simulink model "HVModAL_Fahrzeugmodell"  (R2015b)
settings: Solver=ode1  StartTime=0  StopTime=drp.driving_cycle.tstop  FixedStep=sim_params.Ts  RelTol=1e-5
PreLoadFcn:
  | % Add paths
  | addpath data
  | addpath(genpath('library'))
StartFcn:
  | Simulation.StartTime = tic;
StopFcn:
  | Simulation.DurationTime = toc(Simulation.StartTime);
undefined symbols (not defined in the file or in its folder): Batteries, BMS, BMS_Bat_, C_Nenn_DCDC1, C_Nenn_DCDC2, d2d, DC, DCDC_Converter_efficiency, DcDc_Converters, Dcl, drp, drv, elm, gen, gin, Hdc, hdc, HV, hvb, Hvb, ice, ldc, lib_dcl, lib_hdc, lib_hvb, lib_veh, Link, lossestable, mask_LUT_OCV, mask_LUT_OCV_SOC, mask_LUT_OCV_Temperature, mask_LUT_R, mask_LUT_Rs, mask_LUT_Rs_SOC, mask_LUT_Rs_Temperature, sim_params, speedvec, torquevec, tri, veh, Veh, Vehicle_Chassis
libraries: simulink x29, lib_tri_modules x7, lib_hdc_module x5, lib_gearbox x4, lib_hvb_battery_pack x3, cstblocks x3, PowerLimitBlock x2, MultiCellLibrary x2, lib_aux x1, lib_drv x1, lib_gen x1, lib_elm x1
(part 2 of 7)

== system HVModAL_Fahrzeugmodell/Visualization (Vis) ==
  note: Block Data
  note: Overview
  note: Extended Scopes
  Model Info : simulink/Model-Wide Utilities/Model Info  Frame=on  DisplayStringWithTags=|  HorizontalTextAlignment=Center  LeftAlignmentValue=0.5  SourceBlockDiagram=HVModAL_Fahrzeugmodell  TagMaxNumber=20
      | Last modified
      | %<LastModificationDate>
      | 
      | Model Version
      | %<ModelVersion>
  Show Extended Scope on/off : Constant  Value=sim_params.showextendedscopes
  Speed : Subsystem
  Speed Scope : Scope  NumInputPorts=3
  Subsystem1 : Subsystem
  wires:
  Speed/2(v_actual(km/h)) -> Speed Scope/2  "v_actual(km/h)"
  Speed/1(v_cycle(km/h)) -> Speed Scope/1  "v_cycle(km/h)"
  Speed/3(v_deviation(km/h)) -> Speed Scope/3  "v_deviation(km/h)"
  Show Extended Scope on/off/1 -> ?

== system HVModAL_Fahrzeugmodell/DC-Link (Dcl)/Dcl Voltage Calculation ==
  P : Inport
  Sum of Elements1 : Sum  Inputs=+  SaturateOnIntegerOverflow=on
  Terminator : Terminator
  Dcl_U : Outport
  wires:
  [Dcl_U] -> Sum of Elements1/1
  P/1 -> Terminator/1
  Sum of Elements1/1 -> Dcl_U/1

== system HVModAL_Fahrzeugmodell/Energy Manager (Emg)/Aux Control ==
  Tri_BusPW : Inport
  Hdc_BusPW : Inport  Port=2
  Hvb_BusPW : Inport  Port=3
  Tri_BusSW : Inport  Port=4
  Bus Creator1 : BusCreator  Inputs=3
  Bus Selector : BusSelector  OutputSignals=Tri_P_losses_vec
  Bus Selector1 : BusSelector  OutputSignals=PB_Bat1.Total_Dissipation_Power_W,PB_Bat2.Total_Dissipation_Power_W,PB_Bat3.Total_Dissipation_Power_W,PB_Bat4.Total_Dissipation_Power_W,PB_Bat5.Total_Dissipation_Power_W
  Bus Selector2 : BusSelector  OutputSignals=Hdc_P_losses_vec
  Bus Selector3 : BusSelector  OutputSignals=Elm_P_losses_vec
  Emg_auxControl_hvac : Constant  Value=0
  Emg_auxControl_permanentLoad : Constant
  Sum : Sum  Inputs=++++
  Sum of Elements : Sum  Inputs=+
  Sum of Elements1 : Sum  Inputs=+
  Sum of Elements2 : Sum  Inputs=+
  Sum1 : Sum  Inputs=+++++
  Unit Delay : UnitDelay  SampleTime=sim_params.Ts
  Emg_auxControl_BusSW : Outport
  wires:
  Bus Creator1/1 -> Emg_auxControl_BusSW/1  "Emg_auxControl_BusSW"
  Emg_auxControl_permanentLoad/1 -> Bus Creator1/1  "Emg_auxControl_permanentLoad"
  Emg_auxControl_hvac/1 -> Bus Creator1/2  "Emg_auxControl_hvac"
  Tri_BusPW/1 -> Bus Selector/1
  Hdc_BusPW/1 -> Bus Selector2/1
  Hvb_BusPW/1 -> Bus Selector1/1
  Tri_BusSW/1 -> Bus Selector3/1
  Bus Selector/1 -> Sum of Elements/1  "<Tri_P_losses_vec>"
  Bus Selector2/1 -> Sum of Elements1/1  "<Hdc_P_losses_vec>"
  Bus Selector3/1 -> Sum of Elements2/1  "<Elm_P_losses_vec>"
  Sum/1 -> Unit Delay/1
  Unit Delay/1 -> Bus Creator1/3  "Emg_Cooling_demand"
  Sum of Elements/1 -> Sum/1
  Sum of Elements1/1 -> Sum/3
  Bus Selector1/1 -> Sum1/1  "<Total_Dissipation_Power_W>"
  Bus Selector1/2 -> Sum1/2  "<Total_Dissipation_Power_W>"
  Bus Selector1/3 -> Sum1/3  "<Total_Dissipation_Power_W>"
  Bus Selector1/5 -> Sum1/5  "<Total_Dissipation_Power_W>"
  Bus Selector1/4 -> Sum1/4  "<Total_Dissipation_Power_W>"
  Sum1/1 -> Sum/2
  Sum of Elements2/1 -> Sum/4

== system HVModAL_Fahrzeugmodell/Energy Manager (Emg)/Battery Control ==
  note: 1/100
  Hvb_BusSW : Inport
  Veh_BusSW : Inport  Port=2
  Tri_BusSW : Inport  Port=3
  "Aux_BusSW " : Inport  Port=4
  Bus Selector : BusSelector  OutputSignals=SB_Bat1,SB_Bat2,SB_Bat3
  Bus Selector1 : BusSelector  OutputSignals=Veh_v_actual
  Constant : Constant
  Demux : Demux  Outputs=3
  Driving_Mode : Subsystem
  Emg_fac_Battery4 : Constant  Value=0
  Emg_fac_Battery5 : Constant  Value=0
  Gain : Gain
  Gain1 : Gain  Gain=1/100
  Mux : Mux  Inputs=5
  Sum of Elements : Sum  Inputs=+
  Sum of Elements1 : Sum  Inputs=+
  Sum of Elements2 : Sum  Inputs=+
  Emg_fac_powerDistribution_vec : Outport
  case : Outport  Port=2
  I_rex : Outport  Port=3
  wires:
  Mux/1 -> Emg_fac_powerDistribution_vec/1  "Emg_fac_powerDistribution_vec"
  Emg_fac_Battery4/1 -> Mux/4
  Emg_fac_Battery5/1 -> Mux/5
  Hvb_BusSW/1 -> Bus Selector/1
  Bus Selector/1 -> Driving_Mode/1(SB_BMS_1)  "<SB_Bat1>"
  Bus Selector/2 -> Driving_Mode/2(SB_BMS_2)  "<SB_Bat2>"
  Bus Selector/3 -> Driving_Mode/3(SB_BMS_3)  "<SB_Bat3>"
  Constant/1 -> Driving_Mode/Enable
  Demux/3 -> Sum of Elements2/1
  Demux/2 -> Sum of Elements1/1
  Demux/1 -> Sum of Elements/1
  Gain/1 -> Demux/1
  Driving_Mode/1(vector_PowerDistribution) -> Gain/1
  Sum of Elements/1 -> Mux/1
  Sum of Elements1/1 -> Mux/2
  Sum of Elements2/1 -> Mux/3
  Driving_Mode/2(case) -> case/1
  Veh_BusSW/1 -> Bus Selector1/1
  Bus Selector1/1 -> Driving_Mode/4(Veh_v_actual)  "<Veh_v_actual>"
  Driving_Mode/3(I_rex) -> I_rex/1
  Tri_BusSW/1 -> Driving_Mode/5(Tri_BusSW)
  "Aux_BusSW "/1 -> Driving_Mode/6("Aux_BusSW ")

== system HVModAL_Fahrzeugmodell/Energy Manager (Emg)/Battery Control1 ==
  Hvb_BusSW : Inport
  Battery Control_sfcn : S-Function  FunctionName=Battery_sf  SFunctionModules=""  SFunctionDeploymentMode=off  EnableBusSupport=off  mask{rtw_sf_name=Battery_sf, showVar=off}
      mask prompts: rtw_sf_name "Simulink:masks:GenSFuncName_MP"; showVar "Simulink:masks:GenSFuncShowModuleList_MP"
      mask help: Simulink:masks:GenSFuncDesc_MD
      mask init:
      | displist = '';
      | if ~strcmp(get_param(gcb, 'FunctionName'), rtw_sf_name);
      |   set_param(gcb, 'FunctionName', rtw_sf_name);
      | end
      | % Check if we are generating code
      | rtw_mode = false;
      | if strcmpi(get_param(bdroot(gcb),'SimulationStatus'),'Initializing')
      | 	rtw_mode = strcmpi(get_param(bdroot(gcb),'BuildingRTWCode'),'on') && ...
      | 		~strcmpi(get_param(bdroot(gcb),'TargetStyle'),'SimulationTarget');
      | end
      | if showVar || rtw_mode
      | 	if exist('rtwsfunc') == 2 | exist('rtwsfunc') == 6
      | 		tmplist = rtwsfunc(rtw_sf_name,gcb);
      | 		tmplist = DAStudio.message('Simulink:masks:GenSFuncListOfModules_IC', tmplist);
      | 	elseif showVar
      | 		tmplist1 = DAStudio.message('Simulink:masks:GenSFuncListOfModules_IC', '');
      |         tmplist2 = DAStudio.message('Simulink:masks:GenSFuncNotLicensed_IC');
      |         tmplist = [tmplist1 tmplist2];
      |  	end
      | end
      | if showVar
      |   displist = tmplist;
      | end
      settings: CopyFcn=|
      | if ~strcmp(get_param(gcb,'Linkstatus'),'none') && ...
      | ~strcmp(get_param(gcb,'Linkstatus'),'implicit')
      |   set_param(gcb,'LinkStatus','none');
      | end
      mask Help: eval('feval(''rtwprivate'',''rtwhelpview'',''rtw_sfcn_block'')');
      mask Display:
      | port_label('input',1,'V_Stackvoltage_V');
      | port_label('input',2,'SOC_perc');
      | port_label('input',3,'t_max_currentPower_s');
      | port_label('input',4,'P_max_charge_10s_W');
      | port_label('input',5,'P_max_discharge_10s_W');
      | port_label('input',6,'P_max_charge_30s_W');
      | port_label('input',7,'P_max_discharge_30s_W');
      | port_label('input',8,'b_Bat_available_b');
      | port_label('input',9,'n_bat_type_ID_i');
      | port_label('input',10,'P_currentPower_W');
      | port_label('input',11,'Ri_Bat_eq');
      | port_label('input',12,'Pack_OCV');
      | port_label('input',13,'I_Bat_A');
      | port_label('input',14,'T_Cell_avg');
      | port_label('input',15,'V_Stackvoltage_Vb');
      | port_label('input',16,'SOC_percb');
      | port_label('input',17,'t_max_currentPower_sb');
      | port_label('input',18,'P_max_charge_10s_Wb');
      | port_label('input',19,'P_max_discharge_10s_Wb');
      | port_label('input',20,'P_max_charge_30s_Wb');
      | port_label('input',21,'P_max_discharge_30s_Wb');
      | port_label('input',22,'b_Bat_available_bb');
      | port_label('input',23,'n_bat_type_ID_ib');
      | port_label('input',24,'P_currentPower_Wb');
      | port_label('input',25,'Ri_Bat_eqb');
      | port_label('input',26,'Pack_OCVb');
      | port_label('input',27,'I_Bat_Ab');
      | port_label('input',28,'T_Cell_avgb');
      | port_label('input',29,'V_Stackvoltage_Va');
      | port_label('input',30,'SOC_perca');
      | port_label('input',31,'t_max_currentPower_sa');
      | port_label('input',32,'P_max_charge_10s_Wa');
      | port_label('input',33,'P_max_discharge_10s_Wa');
      | port_label('input',34,'P_max_charge_30s_Wa');
      | port_label('input',35,'P_max_discharge_30s_Wa');
      | port_label('input',36,'b_Bat_available_ba');
      | port_label('input',37,'n_bat_type_ID_ia');
      | port_label('input',38,'P_currentPower_Wa');
      | port_label('input',39,'Ri_Bat_eqa');
      | port_label('input',40,'Pack_OCVa');
      | port_label('input',41,'I_Bat_Aa');
      | port_label('input',42,'T_Cell_avga');
      | port_label('input',43,'V_Stackvoltage_Vc');
      | port_label('input',44,'SOC_percc');
      | port_label('input',45,'t_max_currentPower_sc');
      | port_label('input',46,'P_max_charge_10s_Wc');
      | port_label('input',47,'P_max_discharge_10s_Wc');
      | port_label('input',48,'P_max_charge_30s_Wc');
      | port_label('input',49,'P_max_discharge_30s_Wc');
      | port_label('input',50,'b_Bat_available_bc');
      | port_label('input',51,'n_bat_type_ID_ic');
      | port_label('input',52,'P_currentPower_Wc');
      | port_label('input',53,'Ri_Bat_eqc');
      | port_label('input',54,'Pack_OCVc');
      | port_label('input',55,'I_Bat_Ac');
      | port_label('input',56,'T_Cell_avgc');
      | port_label('input',57,'V_Stackvoltage_Vd');
      | port_label('input',58,'SOC_percd');
      | port_label('input',59,'t_max_currentPower_sd');
      | port_label('input',60,'P_max_charge_10s_Wd');
      | port_label('input',61,'P_max_discharge_10s_Wd');
      | port_label('input',62,'P_max_charge_30s_Wd');
      | port_label('input',63,'P_max_discharge_30s_Wd');
      | port_label('input',64,'b_Bat_available_bd');
      | port_label('input',65,'n_bat_type_ID_id');
      | port_label('input',66,'P_currentPower_Wd');
      | port_label('input',67,'Ri_Bat_eqd');
      | port_label('input',68,'Pack_OCVd');
      | port_label('input',69,'I_Bat_Ad');
      | port_label('input',70,'T_Cell_avgd');
      | port_label('output',1,'Emg_fac_powerDistribution_vec');
  __InputSSForSFun__ : Subsystem
      settings: PermitHierarchicalResolution=ParametersOnly
  __OutputSSForSFun__ : Subsystem
      settings: PermitHierarchicalResolution=ParametersOnly
  Emg_fac_powerDistribution_vec : Outport
  wires:
  Hvb_BusSW/1 -> __InputSSForSFun__/1(Hvb_BusSW)
  __InputSSForSFun__/1(__UniqueOutportName__1__) -> Battery Control_sfcn/1
  __InputSSForSFun__/2(__UniqueOutportName__2__) -> Battery Control_sfcn/2
  __InputSSForSFun__/3(__UniqueOutportName__3__) -> Battery Control_sfcn/3
  __InputSSForSFun__/4(__UniqueOutportName__4__) -> Battery Control_sfcn/4
  __InputSSForSFun__/5(__UniqueOutportName__5__) -> Battery Control_sfcn/5
  __InputSSForSFun__/6(__UniqueOutportName__6__) -> Battery Control_sfcn/6
  __InputSSForSFun__/7(__UniqueOutportName__7__) -> Battery Control_sfcn/7
  __InputSSForSFun__/8(__UniqueOutportName__8__) -> Battery Control_sfcn/8
  __InputSSForSFun__/9(__UniqueOutportName__9__) -> Battery Control_sfcn/9
  __InputSSForSFun__/10(__UniqueOutportName__10__) -> Battery Control_sfcn/10
  __InputSSForSFun__/11(__UniqueOutportName__11__) -> Battery Control_sfcn/11
  __InputSSForSFun__/12(__UniqueOutportName__12__) -> Battery Control_sfcn/12
  __InputSSForSFun__/13(__UniqueOutportName__13__) -> Battery Control_sfcn/13
  __InputSSForSFun__/14(__UniqueOutportName__14__) -> Battery Control_sfcn/14
  __InputSSForSFun__/15(__UniqueOutportName__15__) -> Battery Control_sfcn/15
  __InputSSForSFun__/16(__UniqueOutportName__16__) -> Battery Control_sfcn/16
  __InputSSForSFun__/17(__UniqueOutportName__17__) -> Battery Control_sfcn/17
  __InputSSForSFun__/18(__UniqueOutportName__18__) -> Battery Control_sfcn/18
  __InputSSForSFun__/19(__UniqueOutportName__19__) -> Battery Control_sfcn/19
  __InputSSForSFun__/20(__UniqueOutportName__20__) -> Battery Control_sfcn/20
  __InputSSForSFun__/21(__UniqueOutportName__21__) -> Battery Control_sfcn/21
  __InputSSForSFun__/22(__UniqueOutportName__22__) -> Battery Control_sfcn/22
  __InputSSForSFun__/23(__UniqueOutportName__23__) -> Battery Control_sfcn/23
  __InputSSForSFun__/24(__UniqueOutportName__24__) -> Battery Control_sfcn/24
  __InputSSForSFun__/25(__UniqueOutportName__25__) -> Battery Control_sfcn/25
  __InputSSForSFun__/26(__UniqueOutportName__26__) -> Battery Control_sfcn/26
  __InputSSForSFun__/27(__UniqueOutportName__27__) -> Battery Control_sfcn/27
  __InputSSForSFun__/28(__UniqueOutportName__28__) -> Battery Control_sfcn/28
  __InputSSForSFun__/29(__UniqueOutportName__29__) -> Battery Control_sfcn/29
  __InputSSForSFun__/30(__UniqueOutportName__30__) -> Battery Control_sfcn/30
  __InputSSForSFun__/31(__UniqueOutportName__31__) -> Battery Control_sfcn/31
  __InputSSForSFun__/32(__UniqueOutportName__32__) -> Battery Control_sfcn/32
  __InputSSForSFun__/33(__UniqueOutportName__33__) -> Battery Control_sfcn/33
  __InputSSForSFun__/34(__UniqueOutportName__34__) -> Battery Control_sfcn/34
  __InputSSForSFun__/35(__UniqueOutportName__35__) -> Battery Control_sfcn/35
  __InputSSForSFun__/36(__UniqueOutportName__36__) -> Battery Control_sfcn/36
  __InputSSForSFun__/37(__UniqueOutportName__37__) -> Battery Control_sfcn/37
  __InputSSForSFun__/38(__UniqueOutportName__38__) -> Battery Control_sfcn/38
  __InputSSForSFun__/39(__UniqueOutportName__39__) -> Battery Control_sfcn/39
  __InputSSForSFun__/40(__UniqueOutportName__40__) -> Battery Control_sfcn/40
  __InputSSForSFun__/41(__UniqueOutportName__41__) -> Battery Control_sfcn/41
  __InputSSForSFun__/42(__UniqueOutportName__42__) -> Battery Control_sfcn/42
  __InputSSForSFun__/43(__UniqueOutportName__43__) -> Battery Control_sfcn/43
  __InputSSForSFun__/44(__UniqueOutportName__44__) -> Battery Control_sfcn/44
  __InputSSForSFun__/45(__UniqueOutportName__45__) -> Battery Control_sfcn/45
  __InputSSForSFun__/46(__UniqueOutportName__46__) -> Battery Control_sfcn/46
  __InputSSForSFun__/47(__UniqueOutportName__47__) -> Battery Control_sfcn/47
  __InputSSForSFun__/48(__UniqueOutportName__48__) -> Battery Control_sfcn/48
  __InputSSForSFun__/49(__UniqueOutportName__49__) -> Battery Control_sfcn/49
  __InputSSForSFun__/50(__UniqueOutportName__50__) -> Battery Control_sfcn/50
  __InputSSForSFun__/51(__UniqueOutportName__51__) -> Battery Control_sfcn/51
  __InputSSForSFun__/52(__UniqueOutportName__52__) -> Battery Control_sfcn/52
  __InputSSForSFun__/53(__UniqueOutportName__53__) -> Battery Control_sfcn/53
  __InputSSForSFun__/54(__UniqueOutportName__54__) -> Battery Control_sfcn/54
  __InputSSForSFun__/55(__UniqueOutportName__55__) -> Battery Control_sfcn/55
  __InputSSForSFun__/56(__UniqueOutportName__56__) -> Battery Control_sfcn/56
  __InputSSForSFun__/57(__UniqueOutportName__57__) -> Battery Control_sfcn/57
  __InputSSForSFun__/58(__UniqueOutportName__58__) -> Battery Control_sfcn/58
  __InputSSForSFun__/59(__UniqueOutportName__59__) -> Battery Control_sfcn/59
  __InputSSForSFun__/60(__UniqueOutportName__60__) -> Battery Control_sfcn/60
  __InputSSForSFun__/61(__UniqueOutportName__61__) -> Battery Control_sfcn/61
  __InputSSForSFun__/62(__UniqueOutportName__62__) -> Battery Control_sfcn/62
  __InputSSForSFun__/63(__UniqueOutportName__63__) -> Battery Control_sfcn/63
  __InputSSForSFun__/64(__UniqueOutportName__64__) -> Battery Control_sfcn/64
  __InputSSForSFun__/65(__UniqueOutportName__65__) -> Battery Control_sfcn/65
  __InputSSForSFun__/66(__UniqueOutportName__66__) -> Battery Control_sfcn/66
  __InputSSForSFun__/67(__UniqueOutportName__67__) -> Battery Control_sfcn/67
  __InputSSForSFun__/68(__UniqueOutportName__68__) -> Battery Control_sfcn/68
  __InputSSForSFun__/69(__UniqueOutportName__69__) -> Battery Control_sfcn/69
  __InputSSForSFun__/70(__UniqueOutportName__70__) -> Battery Control_sfcn/70
  Battery Control_sfcn/1 -> __OutputSSForSFun__/1(__UniqueInportName__1__)
  __OutputSSForSFun__/1(Emg_fac_powerDistribution_vec) -> Emg_fac_powerDistribution_vec/1

== system HVModAL_Fahrzeugmodell/Energy Manager (Emg)/Range Extender Control ==
  Ice_BusSW : Inport
  Gin_BusSW : Inport  Port=2
  Emg_fac_genDemand : Constant  Value=0.1
  Terminator6 : Terminator
  Terminator7 : Terminator
  Emg_fac_GenDeman : Outport
  wires:
  Emg_fac_genDemand/1 -> Emg_fac_GenDeman/1  "Emg_auxControl_BusSW"
  Ice_BusSW/1 -> Terminator6/1
  Gin_BusSW/1 -> Terminator7/1

== system HVModAL_Fahrzeugmodell/HV-Batteries (Hvb)/Bat_1 ==
  note: das hier kann eine Parallelschaltung sein
      | immer nur eine Zelle seriell
  note: positive: charge;
      | negative: discharge.
  P_Bat_W : Inport
  T_ambient : Inport  Port=2
  Enable : EnablePort
  Add : Sum
  BMS_Bat_ : Subsystem  AncestorBlock=BMS/BMS_Bat_  mask{mask_b_bat_available_b=mask_b_Bat_Avail, mask_n_bat_type_ID_i=mask_n_BatteryType, mask_f_C_nom_cell=mask_f_C_nom, mask_n_Cell_serial=mask_Num_Zellen_el_ser, mask_n_Cell_parallel=mask_Num_Zellen_el_par, mask_U_Cell_nom=mask_U_Nenn, mask_I_max_cha=mask_I_max_cha, mask_I_max_disch=mask_I_max_disch, mask_v_Radial_Fan=mask_v_Radial_Fan}
      mask prompts: mask_b_bat_available_b "Battery Available"; mask_n_bat_type_ID_i "Battery Tpe ID"; mask_f_C_nom_cell "C nominal"; mask_n_Cell_serial "n Cells serial"; mask_n_Cell_parallel "c Cells parallel"; mask_U_Cell_nom "U Nominal Cellvoltage"; mask_I_max_cha "I max charge cell in A"; mask_I_max_disch "I max discharge cell in A"; mask_v_Radial_Fan "v Radial Fan"
  Battery_Multicell El : MultiCellLibrary/Battery_MultiCell_El  Tag=Battery_Multicell
  Bus Selector : BusSelector  OutputSignals="Forced Air Cooling on,Forced Cooled Coolant Cooling on,Active Heating on,Compressor  Power Factor,Velocity Air"
  Bus Selector2 : BusSelector  OutputSignals=Total_Voltage_V,Total_Current_A,SOC_Vector_Percent,Total_Dissipation_Power_W,Voltage_Vector_V
  Bus Creator1 : BusCreator  Inputs=7
  Cell2ParallelCells : Gain  Gain=mask_Num_Zellen_el_par
  Delay : Delay  DelayLength=1  InitialCondition=0
  Gain1 : Gain  Gain=-1
  Gain2 : Gain  Gain=0
  MinMax : MinMax  Function=max
  P_cellsParallel2I_cellsParallel : Product  Inputs=/*
  ParallelCells2Pack : Gain  Gain=mask_Num_Zellen_el_ser
  Temp_model : Subsystem
  Unit Delay : UnitDelay  InitialCondition=mask_U_Nenn*mask_Num_Zellen_el_ser  SampleTime=-1
  cell 2 pack1 : Gain  Gain=mask_Num_Zellen_el_ser*mask_Num_Zellen_el_par
  pack2parallel_cells : Gain  Gain=1/mask_Num_Zellen_el_ser
  parallel2cell : Gain  Gain=1/mask_Num_Zellen_el_par
  PB_Bat : Outport
  SB_Bat : Outport  Port=2
  wires:
  Battery_Multicell El/1 -> Bus Selector2/1
  P_cellsParallel2I_cellsParallel/1 -> parallel2cell/1
  Unit Delay/1 -> P_cellsParallel2I_cellsParallel/1
  Bus Selector2/1 -> Unit Delay/1, ParallelCells2Pack/1  "<Total_Voltage_V>"
  Bus Selector2/3 -> MinMax/1  "<SOC_Vector_Percent>"
  Bus Selector2/2 -> Cell2ParallelCells/1  "<Total_Current_A>"
  Bus Selector2/4 -> cell 2 pack1/1, Temp_model/1(Q_dotLoss)  "<Total_Dissipation_Power_W>"
  cell 2 pack1/1 -> Bus Creator1/4  "Total_Dissipation_Power_W"
  MinMax/1 -> Bus Creator1/3  "SOC_Vector_Percent"
  Bus Selector2/5 -> Gain2/1, Bus Creator1/5  "<Voltage_Vector_V>"
  Gain2/1 -> Add/1
  Add/1 -> Delay/1
  Delay/1 -> Bus Creator1/6, Battery_Multicell El/2  "T_cell_degC"
  ParallelCells2Pack/1 -> Bus Creator1/1  "Total_Voltage_V"
  pack2parallel_cells/1 -> P_cellsParallel2I_cellsParallel/2
  Bus Creator1/1 -> BMS_Bat_/1(PB_Bat), PB_Bat/1
  parallel2cell/1 -> Gain1/1
  Cell2ParallelCells/1 -> Bus Creator1/2  "Total_Current_A"
  T_ambient/1 -> Temp_model/2(T_environment)
  BMS_Bat_/1(SB_BMS) -> Bus Selector/1, SB_Bat/1
  Bus Selector/1 -> Temp_model/3(ForcedAir Cooling on)  "<Forced Air Cooling on>"
  Temp_model/1(T_cell  avg) -> Add/2  "T_cell avg"
  Bus Selector/3 -> Temp_model/5(Active Heating on)  "<Active Heating on>"
  Bus Selector/4 -> Temp_model/6(Compressor Power Factor)  "<Compressor  Power Factor>"
  P_Bat_W/1 -> pack2parallel_cells/1
  Bus Selector/5 -> Temp_model/7(Velocity Airstream)  "<Velocity Air>"
  Gain1/1 -> Battery_Multicell El/1
  Bus Selector/2 -> Temp_model/4(Forced Cooled Coolant Cooling on)  "<Forced Cooled Coolant Cooling on>"
  Temp_model/2(Q_dot_ AllCompressors +PTC) -> Bus Creator1/7  "P_T_control_power_W"

== system HVModAL_Fahrzeugmodell/HV-Batteries (Hvb)/Bat_2 ==
  note: das hier kann eine Parallelschaltung sein
      | immer nur eine Zelle seriell
  note: positive: charge;
      | negative: discharge.
  P_Bat_W : Inport
  T_ambient : Inport  Port=2
  Enable : EnablePort
  Add : Sum
  BMS_Bat_ : Subsystem  AncestorBlock=BMS/BMS_Bat_  mask{mask_b_bat_available_b=mask_b_Bat_Avail, mask_n_bat_type_ID_i=mask_n_BatteryType, mask_f_C_nom_cell=mask_f_C_nom, mask_n_Cell_serial=mask_Num_Zellen_el_ser, mask_n_Cell_parallel=mask_Num_Zellen_el_par, mask_U_Cell_nom=mask_U_Nenn, mask_I_max_cha=mask_I_max_cha, mask_I_max_disch=mask_I_max_disch, mask_v_Radial_Fan=mask_v_Radial_Fan}
      mask prompts: mask_b_bat_available_b "Battery Available"; mask_n_bat_type_ID_i "Battery Tpe ID"; mask_f_C_nom_cell "C nominal"; mask_n_Cell_serial "n Cells serial"; mask_n_Cell_parallel "c Cells parallel"; mask_U_Cell_nom "U Nominal Cellvoltage"; mask_I_max_cha "I max charge cell in A"; mask_I_max_disch "I max discharge cell in A"; mask_v_Radial_Fan "v Radial Fan"
  Battery_Multicell El : MultiCellLibrary/Battery_MultiCell_El  Tag=Battery_Multicell
  Bus Selector : BusSelector  OutputSignals="Forced Air Cooling on,Forced Cooled Coolant Cooling on,Active Heating on,Compressor  Power Factor,Velocity Air"
  Bus Selector2 : BusSelector  OutputSignals=Total_Voltage_V,Total_Current_A,SOC_Vector_Percent,Total_Dissipation_Power_W,Voltage_Vector_V
  Bus Creator1 : BusCreator  Inputs=7
  Cell2ParallelCells : Gain  Gain=mask_Num_Zellen_el_par
  Delay : Delay  DelayLength=1  InitialCondition=0
  Gain1 : Gain  Gain=-1
  Gain2 : Gain  Gain=0
  MinMax : MinMax  Function=max
  P_cellsParallel2I_cellsParallel : Product  Inputs=/*
  ParallelCells2Pack : Gain  Gain=mask_Num_Zellen_el_ser
  Saturation : Saturate  UpperLimit=hvb.Bat2.P_max_disch  LowerLimit=hvb.Bat2.P_max_cha
  Temp_model : Subsystem
  Unit Delay : UnitDelay  InitialCondition=mask_U_Nenn*mask_Num_Zellen_el_ser  SampleTime=-1
  cell 2 pack1 : Gain  Gain=mask_Num_Zellen_el_ser*mask_Num_Zellen_el_par
  pack2parallel_cells : Gain  Gain=1/mask_Num_Zellen_el_ser
  parallel2cell : Gain  Gain=1/mask_Num_Zellen_el_par
  PB_Bat : Outport
  SB_Bat : Outport  Port=2
  wires:
  Battery_Multicell El/1 -> Bus Selector2/1
  P_cellsParallel2I_cellsParallel/1 -> parallel2cell/1
  Unit Delay/1 -> P_cellsParallel2I_cellsParallel/1
  Bus Selector2/1 -> Unit Delay/1, ParallelCells2Pack/1  "<Total_Voltage_V>"
  Bus Selector2/3 -> MinMax/1  "<SOC_Vector_Percent>"
  Bus Selector2/2 -> Cell2ParallelCells/1  "<Total_Current_A>"
  Bus Selector2/4 -> cell 2 pack1/1, Temp_model/1(Q_dotLoss)  "<Total_Dissipation_Power_W>"
  cell 2 pack1/1 -> Bus Creator1/4  "Total_Dissipation_Power_W"
  MinMax/1 -> Bus Creator1/3  "SOC_Vector_Percent"
  Bus Selector2/5 -> Gain2/1, Bus Creator1/5  "<Voltage_Vector_V>"
  Gain2/1 -> Add/1
  Add/1 -> Delay/1
  Delay/1 -> Bus Creator1/6, Battery_Multicell El/2  "T_cell_degC"
  ParallelCells2Pack/1 -> Bus Creator1/1  "Total_Voltage_V"
  pack2parallel_cells/1 -> P_cellsParallel2I_cellsParallel/2
  Bus Creator1/1 -> BMS_Bat_/1(PB_Bat), PB_Bat/1
  parallel2cell/1 -> Gain1/1
  Cell2ParallelCells/1 -> Bus Creator1/2  "Total_Current_A"
  T_ambient/1 -> Temp_model/2(T_environment)
  BMS_Bat_/1(SB_BMS) -> Bus Selector/1, SB_Bat/1
  Bus Selector/1 -> Temp_model/3(ForcedAir Cooling on)  "<Forced Air Cooling on>"
  Temp_model/1(T_cell  avg) -> Add/2  "T_cell avg"
  Bus Selector/3 -> Temp_model/5(Active Heating on)  "<Active Heating on>"
  Bus Selector/4 -> Temp_model/6(Compressor Power Factor)  "<Compressor  Power Factor>"
  Bus Selector/5 -> Temp_model/7(Velocity Airstream)  "<Velocity Air>"
  Gain1/1 -> Battery_Multicell El/1
  Bus Selector/2 -> Temp_model/4(Forced Cooled Coolant Cooling on)  "<Forced Cooled Coolant Cooling on>"
  Temp_model/2(Q_dot_ AllCompressors +PTC) -> Bus Creator1/7  "P_T_control_power_W"
  P_Bat_W/1 -> pack2parallel_cells/1

== system HVModAL_Fahrzeugmodell/HV-DcDc_Converters (Hdc)/Determine DCL_U ==
  U_DCL by Battery : Inport
  U_DCL by String : Inport  Port=2
  Index Vector : MultiPortSwitch  Inputs=1
  Switch : Switch  Criteria=u2 ~= 0
  any Bat direct con. to DCL? : Constant  Value=hdc.flags.lastBatteryConnectedToDCL
  number of batteries : Constant  Value=hdc.num_Bat
  U_DCL : Outport
  wires:
  U_DCL by Battery/1 -> Index Vector/2
  number of batteries/1 -> Index Vector/1
  Switch/1 -> U_DCL/1
  Index Vector/1 -> Switch/1
  U_DCL by String/1 -> Switch/3
  any Bat direct con. to DCL?/1 -> Switch/2

== system HVModAL_Fahrzeugmodell/HV-DcDc_Converters (Hdc)/Determine Hdc_P_max_vec ==
  P_max_DCDC : Inport
  Assignment : Assignment  DiagnosticForDimensions=Warning  IndexOptions=Index vector (port)  Indices=1  OutputSizes=1
  Pmax replace value : Constant  Value=1e6
  Switch : Switch  Criteria=u2 ~= 0
  any Bat direct con. to DCL? : Constant  Value=hdc.flags.lastBatteryConnectedToDCL
  number of batteries : Constant  Value=hdc.num_Bat
  Hdc_P_max_vec : Outport
  wires:
  Assignment/1 -> Switch/1  "Pmax with last value replaced by inf"
  any Bat direct con. to DCL?/1 -> Switch/2
  Switch/1 -> Hdc_P_max_vec/1
  Pmax replace value/1 -> Assignment/2
  number of batteries/1 -> Assignment/3
  P_max_DCDC/1 -> Switch/3, Assignment/1  "Pmax given by DC/DC"

== system HVModAL_Fahrzeugmodell/HV-DcDc_Converters (Hdc)/Determine P_DCL and P_bat ==
  note: P_bat by DCDC is the P_DCL demand plus losses
  P_DCL demand : Inport
  P_bat by DCDC : Inport  Port=2
  Assignment : Assignment  DiagnosticForDimensions=Warning  IndexOptions=Index vector (port)  Indices=1  OutputSizes=1
  Index Vector : MultiPortSwitch  Inputs=1
  Switch : Switch  Criteria=u2 ~= 0
  any Bat direct con. to DCL? : Constant  Value=hdc.flags.lastBatteryConnectedToDCL
  number of batteries : Constant  Value=hdc.num_Bat
  P_bat : Outport
  P_DCL : Outport  Port=2
  wires:
  P_bat by DCDC/1 -> Switch/3, Assignment/1  "P_bat"
  number of batteries/1 -> Assignment/3, Index Vector/1
  P_DCL demand/1 -> P_DCL/1, Index Vector/2
  Index Vector/1 -> Assignment/2  "power demand of last battery"
  Switch/1 -> P_bat/1
  any Bat direct con. to DCL?/1 -> Switch/2
  Assignment/1 -> Switch/1

== system HVModAL_Fahrzeugmodell/HV-DcDc_Converters (Hdc)/HV-DcDc_Converter_Slave ==
  Hvb_U_Bat : Inport
  Emg_U_dcDemand : Inport  Port=2
  Emg_P_dcDemand : Inport  Port=3
  Dcl_U : Inport  Port=4
  case : Inport  Port=5
  Enable : EnablePort
  Abs1 : Abs
  Add : Sum  Inputs=-+
  Add1 : Sum
  Control Unit1 : Subsystem  AncestorBlock=lib_hdc_module/HV-DcDc_Converter_Master/Control Unit1
  Divide : Product  Inputs=*/
  Gain : Gain  Gain=0.5
  Saturation : Saturate  UpperLimit=1  LowerLimit=0.1
  Sum : Sum  Inputs=+
  Terminator : Terminator
  Thermal System : lib_hdc_module/HV-DcDc_Converter_Master/Thermal System
  n-D Lookup Table : Lookup_n-D  NumberOfTableDimensions=4  BreakpointsForDimension1=DCDCname.Vin  BreakpointsForDimension2=DCDCname.Vout  BreakpointsForDimension3=DCDCname.Pout  BreakpointsForDimension4=DCDCname.Temperature  Table=DCDCname.EfficiencyMap  InternalRulePriority=Speed  RndMeth=Simplest  InputSameDT=on
  Hdc_P_bat : Outport
  Hdc_fac_eta : Outport  Port=2
  Hdc_P_losses : Outport  Port=3
  Hdc_flg_error : Outport  Port=4
  Hdc_P_dcLink : Outport  Port=5
  at_Junction : Outport  Port=6
  Pmax : Outport  Port=7
  wires:
  Emg_U_dcDemand/1 -> Terminator/1
  Dcl_U/1 -> [U_DCL], n-D Lookup Table/2, Control Unit1/2(Emg_U_dcDemand)
  Add1/1 -> Hdc_P_bat/1
  Hvb_U_Bat/1 -> [U_bat], n-D Lookup Table/1, Control Unit1/4(Emg_U_bat)
  Add/1 -> Hdc_P_losses/1, Add1/1
  n-D Lookup Table/1 -> Saturation/1
  Control Unit1/1(Pdc_avail) -> Hdc_P_dcLink/1, Add1/2, Abs1/1
  Control Unit1/2(Error) -> Hdc_flg_error/1
  Emg_P_dcDemand/1 -> Control Unit1/1(Emg_Pdc_demand)
  Control Unit1/3(Pmax) -> Pmax/1
  Abs1/1 -> Thermal System/3, n-D Lookup Table/3, Add/1, Divide/1
  Divide/1 -> Add/2
  Saturation/1 -> Hdc_fac_eta/1, Divide/2
  Sum/1 -> Gain/1
  Gain/1 -> n-D Lookup Table/4, at_Junction/1
  Thermal System/1 -> Control Unit1/3(at_Junction), Sum/1
  [U_bat] -> Thermal System/1
  [U_DCL] -> Thermal System/2
  case/1 -> Control Unit1/5(case)

== system HVModAL_Fahrzeugmodell/Sim_Control/Speed ==
  Bus Selector1 : BusSelector  OutputSignals=Drp_v_vehDesired
  Bus Selector2 : BusSelector  OutputSignals=Veh_v_actual
  Gain : Gain  Gain=3.6
  Gain1 : Gain  Gain=3.6
  Sum : Sum  Inputs=+-
  v_cycle(km/h) : Outport
  v_actual(km/h) : Outport  Port=2
  v_deviation(km/h) : Outport  Port=3
  wires:
  Bus Selector2/1 -> Gain/1  "<Veh_v_actual>"
  Bus Selector1/1 -> Gain1/1  "<Drp_v_vehDesired>"
  [Drp_SWBus_toworkspace] -> Bus Selector1/1
  [Veh_SWBus_toworkspace] -> Bus Selector2/1
  Sum/1 -> v_deviation(km/h)/1  "v_deviation(km/h)"
  Gain/1 -> v_actual(km/h)/1, Sum/2  "v_actual(km/h)"
  Gain1/1 -> v_cycle(km/h)/1, Sum/1  "v_cycle(km/h)"

== system HVModAL_Fahrzeugmodell/To Workspace (Two)/Aux ==
  Aux_bus : Outport
  wires:
  [Aux_BusPB_ToLogging] -> Aux_bus/1

== system HVModAL_Fahrzeugmodell/To Workspace (Two)/Data Logging ==
  result_Bus : Inport
  Enable : EnablePort
  To Workspace : ToWorkspace  VariableName=result  SaveFormat=Timeseries  SampleTime=sim_params.Ts
      settings: Decimation=sim_params.logging_decimation
  wires:
  result_Bus/1 -> To Workspace/1

== system HVModAL_Fahrzeugmodell/To Workspace (Two)/Dcl ==
  Bus Creator : BusCreator  Inputs=1
  Dcl bus : Outport
  wires:
  Bus Creator/1 -> Dcl bus/1
  [Dcl_BusPB_toworkspace] -> Bus Creator/1  "PB"

== system HVModAL_Fahrzeugmodell/To Workspace (Two)/Drp ==
  Bus Creator : BusCreator  Inputs=1
  Drp bus : Outport
  wires:
  [Drp_SWBus_toworkspace] -> Bus Creator/1  "SB"
  Bus Creator/1 -> Drp bus/1

== system HVModAL_Fahrzeugmodell/To Workspace (Two)/Elm ==
  Bus Creator : BusCreator  Inputs=1
  Bus Creator1 : BusCreator  Inputs=1
  Elm bus : Outport
  wires:
  Bus Creator/1 -> Bus Creator1/1
  Bus Creator1/1 -> Elm bus/1
  [Elm_BusPB_toworkspace] -> Bus Creator/1  "PB"

== system HVModAL_Fahrzeugmodell/To Workspace (Two)/Emg ==
  Drp bus : Outport
  wires:
  [EMG_BusSW_ToLogging] -> Drp bus/1

== system HVModAL_Fahrzeugmodell/To Workspace (Two)/Hdc ==
  Bus Creator : BusCreator  Inputs=2
  Hdc bus : Outport
  wires:
  Bus Creator/1 -> Hdc bus/1
  [Hdc_SWBus_toWorkspace] -> Bus Creator/2  "SB"
  [Hdc_PBBus_toWorkspace] -> Bus Creator/1  "PB"

== system HVModAL_Fahrzeugmodell/To Workspace (Two)/Hvb ==
  Bus Creator : BusCreator  Inputs=2
  Hvb_PB : Outport
  wires:
  [Hvb_PBbus_toworkspace] -> Bus Creator/1  "PB"
  [Hvb_SWbus_toworkspace] -> Bus Creator/2  "SB"
  Bus Creator/1 -> Hvb_PB/1  "HVB"

== system HVModAL_Fahrzeugmodell/To Workspace (Two)/Tri ==
  Bus Creator2 : BusCreator  Inputs=2
  Tri bus : Outport
  wires:
  Bus Creator2/1 -> Tri bus/1
  [Tri_BusPB_toWorkspace] -> Bus Creator2/1  "PB"
  [Tri_BusSW_toWorkspace] -> Bus Creator2/2  "SB"

== system HVModAL_Fahrzeugmodell/To Workspace (Two)/Veh ==
  Veh bus : Outport
  wires:
  [Veh_SWBus_toworkspace] -> Veh bus/1

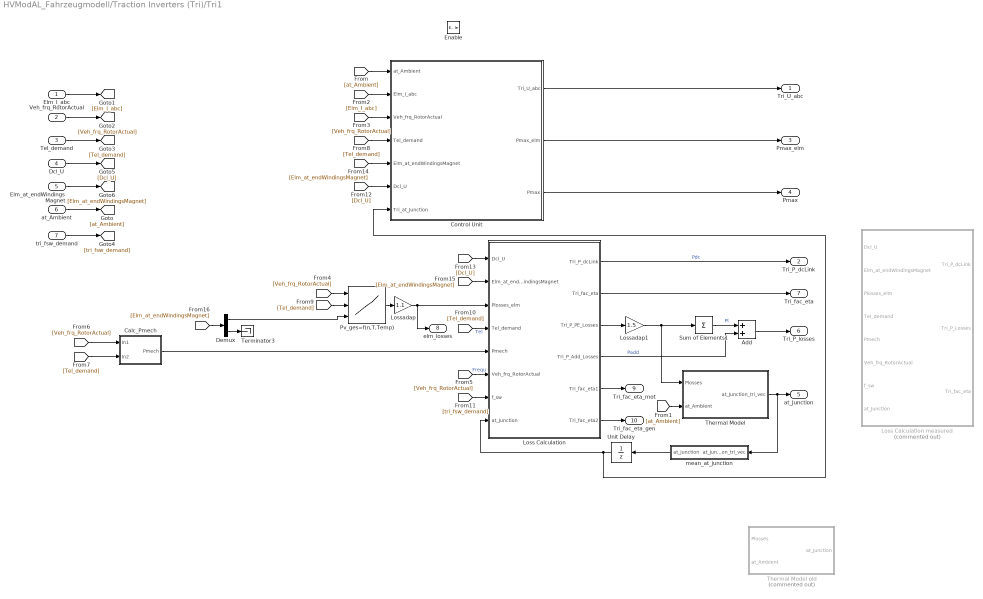
== system HVModAL_Fahrzeugmodell/Traction Inverters (Tri)/Tri1 ==
  Elm_I_abc : Inport
  Veh_frq_RotorActual : Inport  Port=2
  Tel_demand : Inport  Port=3
  Dcl_U : Inport  Port=4
  Elm_at_endWindingsMagnet : Inport  Port=5
  at_Ambient : Inport  Port=6
  tri_fsw_demand : Inport  Port=7
  Enable : EnablePort
  Add : Sum
  Calc_Pmech : Subsystem
  Control Unit : Subsystem
  Demux : Demux  Outputs=2
  Loss Calculation : Subsystem
  Loss Calculation measured : Subsystem  Commented=on
  Lossadap : Gain  Gain=1.1
  Lossadap1 : Gain  Gain=1.5
  Pv_ges=f(n,T,Temp) : Lookup_n-D  NumberOfTableDimensions=3  BreakpointsForDimension1=ELMname.n/60  BreakpointsForDimension2=ELMname.tq  BreakpointsForDimension3=ELMname.temp  Table=ELMname.pwr_loss_total  InternalRulePriority=Speed  RndMeth=Simplest  InputSameDT=on
  Sum of Elements1 : Sum  Inputs=+
  Terminator3 : Terminator
  Thermal Model : Subsystem
  Thermal Model old : Subsystem  Commented=on
  Unit Delay : UnitDelay  InitialCondition=60  SampleTime=-1
  mean_at_junction : Subsystem
  Tri_U_abc : Outport
  Tri_P_dcLink : Outport  Port=2
  Pmax_elm : Outport  Port=3
  Pmax : Outport  Port=4
  at_Junction : Outport  Port=5
  Tri_P_losses : Outport  Port=6
  Tri_fac_eta : Outport  Port=7
  elm_losses : Outport  Port=8
  Tri_fac_eta_mot : Outport  Port=9
  Tri_fac_eta_gen : Outport  Port=10
  wires:
  mean_at_junction/1(at_junction) -> Unit Delay/1
  Loss Calculation/4(Tri_P_Add_Losses) -> Add/2  "Padd"
  Add/1 -> Tri_P_losses/1
  Sum of Elements1/1 -> Add/1  "Pl"
  Elm_at_endWindingsMagnet/1 -> [Elm_at_endWindingsMagnet]
  [Elm_at_endWindingsMagnet] -> Demux/1
  [Elm_at_endWindingsMagnet] -> Loss Calculation/2(Elm_at_endWindingsMagnet)
  [Elm_at_endWindingsMagnet] -> Control Unit/5(Elm_at_endWindingsMagnet)
  Dcl_U/1 -> [Dcl_U]
  [Dcl_U] -> Loss Calculation/1(Dcl_U)
  [Dcl_U] -> Control Unit/6(Dcl_U)
  [Tel_demand] -> Calc_Pmech/2(In2)
  [tri_fsw_demand] -> Loss Calculation/7(f_sw)
  tri_fsw_demand/1 -> [tri_fsw_demand]
  Tel_demand/1 -> [Tel_demand]
  [Tel_demand] -> Loss Calculation/4(Tel_demand)  "Tel"
  [Tel_demand] -> Pv_ges=f(n,T,Temp)/2
  [Tel_demand] -> Control Unit/4(Tel_demand)
  Veh_frq_RotorActual/1 -> [Veh_frq_RotorActual]
  [Veh_frq_RotorActual] -> Calc_Pmech/1(In1)
  [Veh_frq_RotorActual] -> Loss Calculation/6(Veh_frq_RotorActual)  "Frequ"
  [Veh_frq_RotorActual] -> Pv_ges=f(n,T,Temp)/1
  [Veh_frq_RotorActual] -> Control Unit/3(Veh_frq_RotorActual)
  [Elm_I_abc] -> Control Unit/2(Elm_I_abc)
  Elm_I_abc/1 -> [Elm_I_abc]
  [at_Ambient] -> Thermal Model/2(at_Ambient)
  [at_Ambient] -> Control Unit/1(at_Ambient)
  Pv_ges=f(n,T,Temp)/1 -> Lossadap/1
  Control Unit/2(Pmax_elm) -> Pmax_elm/1
  Thermal Model/1(at_Junction_tri_vec) -> at_Junction/1, mean_at_junction/1(at_junction_tri_vec)
  Unit Delay/1 -> Control Unit/7(Tri_at_Junction), Loss Calculation/8(at_Junction)
  at_Ambient/1 -> [at_Ambient]
  Control Unit/3(Pmax) -> Pmax/1
  Control Unit/1(Tri_U_abc) -> Tri_U_abc/1
  Calc_Pmech/1(Pmech) -> Loss Calculation/5(Pmech)
  Loss Calculation/1(Tri_P_dcLink) -> Tri_P_dcLink/1  "Pdc"
  Loss Calculation/2(Tri_fac_eta) -> Tri_fac_eta/1
  Loss Calculation/5(Tri_fac_eta1) -> Tri_fac_eta_mot/1
  Loss Calculation/6(Tri_fac_eta2) -> Tri_fac_eta_gen/1
  Loss Calculation/3(Tri_P_PE_Losses) -> Lossadap1/1
  Lossadap/1 -> Loss Calculation/3(Plosses_elm), elm_losses/1
  Demux/1 -> Pv_ges=f(n,T,Temp)/3
  Demux/2 -> Terminator3/1
  Lossadap1/1 -> Sum of Elements1/1, Thermal Model/1(Plosses)

== system HVModAL_Fahrzeugmodell/Vehicle_Chassis (Veh)/Axle Load ==
  a_actual (m/s^2) : Inport
  grad_cycle (rad) : Inport  Port=2
  CG back Distance : Constant  Value=veh.cg.backdistance
  CG front Distance : Constant  Value=veh.cg.frontdistance
  CG height : Constant  Value=veh.cg.height
  Product{,1..3} (4 alike) : Product  Inputs=/***
  Product4 : Product  Inputs=/**
  Product5 : Product
  Product6 : Product
  Sum : Sum  Inputs=|-+-
  Sum1 : Sum  Inputs=|+++
  Trigonometric Function : Trigonometry  Operator=cos
  Trigonometric Function1 : Trigonometry
  Veh_weight [kg] : Constant  Value=veh.totalweight
  gravity (m/s^2) : Constant  Value=9.81274
  wheel_dictance [m] : Constant  Value=veh.wheel.distance
  front_load [N] : Outport
  back_load [N] : Outport  Port=2
  wires:
  CG back Distance/1 -> Product/2
  grad_cycle (rad)/1 -> Trigonometric Function1/1, Trigonometric Function/1
  Trigonometric Function/1 -> Product1/3, Product/3
  wheel_dictance [m]/1 -> Product4/1, Product3/1, Product1/1, Product/1, Product2/1
  gravity (m/s^2)/1 -> Product3/4, Product1/4, Product2/4, Product/4
  CG front Distance/1 -> Product1/2
  CG height/1 -> Product2/3, Product3/2, Product4/3
  Trigonometric Function1/1 -> Product3/3, Product2/2
  Product/1 -> Sum/2
  Product2/1 -> Sum/1
  Product4/1 -> Sum1/1, Sum/3
  Sum/1 -> Product5/1
  Veh_weight [kg]/1 -> Product6/2, Product5/2
  Sum1/1 -> Product6/1
  Product3/1 -> Sum1/3
  Product1/1 -> Sum1/2
  Product6/1 -> back_load [N]/1
  Product5/1 -> front_load [N]/1
  a_actual (m/s^2)/1 -> Product4/2

== system HVModAL_Fahrzeugmodell/Vehicle_Chassis (Veh)/Calculate Reduced Vehicle Mass ==
  1/r_dyn² : Gain  Gain=1/veh.wheel.radius^2  SaturateOnIntegerOverflow=on  OutDataTypeStr=Inherit: Same as input  ParamDataTypeStr=Inherit: Same as input
  Driver : Constant  Value=drv.driverweight
  Electric Komponents : Sum  Inputs=+++++  SaturateOnIntegerOverflow=on  InputSameDT=on  OutDataTypeStr=Inherit: Same as first input
  Elm : Constant  Value=elm.weight
  Gearbox : Constant  Value=veh.gearbox.weight
  Generator+FI : Constant  Value=gin.weight+gen.weight
  Hdc : Constant  Value=hdc.weight
  Hvb : Constant  Value=hvb.weight
  Hybrid : Sum  SaturateOnIntegerOverflow=on  InputSameDT=on  OutDataTypeStr=Inherit: Same as first input
  ICE : Constant  Value=ice.weight
  Ldc : Constant  Value=ldc.weight
  Motor Inertia1 : Constant  Value=veh.gearbox.gearbox1.motor_inertia
  Motor Inertia2 : Constant  Value=veh.gearbox.gearbox2.motor_inertia
  Motor Inertia3 : Constant  Value=veh.gearbox.gearbox3.motor_inertia
  Motor Inertia4 : Constant  Value=veh.gearbox.gearbox4.motor_inertia
  Sum : Sum  SaturateOnIntegerOverflow=on  InputSameDT=on  OutDataTypeStr=Inherit: Same as first input
  Sum1 : Sum  Inputs=+++  SaturateOnIntegerOverflow=on  InputSameDT=on  OutDataTypeStr=Inherit: Same as first input
  Sum2 : Sum  SaturateOnIntegerOverflow=on  InputSameDT=on  OutDataTypeStr=Inherit: Same as first input
  Sum3 : Sum  Inputs=++++  SaturateOnIntegerOverflow=on  InputSameDT=on  OutDataTypeStr=Inherit: Same as first input
  Sum4 : Sum  Inputs=+++  SaturateOnIntegerOverflow=on  InputSameDT=on  OutDataTypeStr=Inherit: Same as first input
  Tri : Constant  Value=tri.weight
  Vehicle Weight : Constant  Value=veh.weight
  Wheels Inertia : Constant  Value=4*veh.wheel.inertia
  ratio²1 : Gain  Gain=veh.gearbox.gearbox1.ratio^2*elm.elm1.phys_avail  SaturateOnIntegerOverflow=on  OutDataTypeStr=Inherit: Same as input  ParamDataTypeStr=Inherit: Same as input
  ratio²2 : Gain  Gain=veh.gearbox.gearbox2.ratio^2*elm.elm2.phys_avail  SaturateOnIntegerOverflow=on  OutDataTypeStr=Inherit: Same as input  ParamDataTypeStr=Inherit: Same as input
  ratio²3 : Gain  Gain=veh.gearbox.gearbox3.ratio^2*elm.elm3.phys_avail  SaturateOnIntegerOverflow=on  OutDataTypeStr=Inherit: Same as input  ParamDataTypeStr=Inherit: Same as input
  ratio²4 : Gain  Gain=veh.gearbox.gearbox4.ratio^2*elm.elm4.phys_avail  SaturateOnIntegerOverflow=on  OutDataTypeStr=Inherit: Same as input  ParamDataTypeStr=Inherit: Same as input
  m_red(kg) : Outport
  wires:
  Motor Inertia4/1 -> ratio²4/1
  Vehicle Weight/1 -> Sum1/2
  Wheels Inertia/1 -> Sum/2
  ratio²4/1 -> Sum3/4
  Sum/1 -> 1/r_dyn²/1
  1/r_dyn²/1 -> Sum1/1
  Sum1/1 -> Sum2/1
  Electric Komponents/1 -> Sum2/2
  Tri/1 -> Electric Komponents/1
  Hvb/1 -> Electric Komponents/2
  Hdc/1 -> Electric Komponents/3
  Elm/1 -> Electric Komponents/5
  Ldc/1 -> Electric Komponents/4
  Sum2/1 -> Sum4/1
  Gearbox/1 -> Sum1/3
  Generator+FI/1 -> Hybrid/2
  ICE/1 -> Hybrid/1
  Hybrid/1 -> Sum4/2
  Sum4/1 -> m_red(kg)/1
  Driver/1 -> Sum4/3
  ratio²3/1 -> Sum3/3
  Sum3/1 -> Sum/1
  Motor Inertia3/1 -> ratio²3/1
  ratio²2/1 -> Sum3/2
  ratio²1/1 -> Sum3/1
  Motor Inertia2/1 -> ratio²2/1
  Motor Inertia1/1 -> ratio²1/1

== system HVModAL_Fahrzeugmodell/Vehicle_Chassis (Veh)/Drive Shaft ==
  Tin1 : Inport
  Tin2 : Inport  Port=2
  Tin3 : Inport  Port=3
  Tin4 : Inport  Port=4
  1/r_dyn : Gain  Gain=1/veh.wheel.radius  SaturateOnIntegerOverflow=on  OutDataTypeStr=Inherit: Same as input  ParamDataTypeStr=Inherit: Same as input
  Sum : Sum  Inputs=++++
  F_acc(N) : Outport
  tag scope: Twheel_demand_Nm=global
  wires:
  1/r_dyn/1 -> F_acc(N)/1  "F_acc(N)"
  Tin2/1 -> Sum/2
  Tin1/1 -> Sum/1
  Sum/1 -> [Twheel_demand_Nm], 1/r_dyn/1
  Tin3/1 -> Sum/3
  Tin4/1 -> Sum/4

== system HVModAL_Fahrzeugmodell/Vehicle_Chassis (Veh)/Driving Data ==
  m_red [kg] : Inport
  F_drive [N] : Inport  Port=2
  Emg_gearbox_vec : Inport  Port=3
  Calculate Actual Speed : Subsystem
  Conversions : Subsystem
  n_motor(rpm) : Outport
  v_wheel(m/s) : Outport  Port=2
  a_actual [m/s] : Outport  Port=3
  wires:
  Conversions/1(veh_n_motor_vec) -> n_motor(rpm)/1
  m_red [kg]/1 -> Calculate Actual Speed/1(m_red [kg])
  F_drive [N]/1 -> Calculate Actual Speed/2(F_drive [N])
  Calculate Actual Speed/1(v_actual [m/s]) -> Conversions/1(v_actual (m/s)), v_wheel(m/s)/1
  Calculate Actual Speed/2(a_actual [m/s]) -> a_actual [m/s]/1
  Emg_gearbox_vec/1 -> Conversions/2(Emg_gearbox_vec)

== system HVModAL_Fahrzeugmodell/Vehicle_Chassis (Veh)/Driving Forces ==
  F_acc(N) : Inport
  grad_cycle(rad) : Inport  Port=2
  v_actual(m/s) : Inport  Port=3
  Aerodynamic Resistance : Subsystem
  Climbing Resistance : Subsystem
  Rolling Resistance : Subsystem
  Sum1 : Sum  Inputs=+++  SaturateOnIntegerOverflow=on  InputSameDT=on  OutDataTypeStr=Inherit: Same as first input
  Sum2 : Sum  Inputs=-+  SaturateOnIntegerOverflow=on  InputSameDT=on  OutDataTypeStr=Inherit: Same as first input
  F_drive(N) : Outport
  F_aero : Outport  Port=2
  F_roll : Outport  Port=3
  F_climb : Outport  Port=4
  F_acc : Outport  Port=5
  wires:
  F_acc(N)/1 -> F_acc/1, Sum2/2
  grad_cycle(rad)/1 -> Rolling Resistance/2(gradient), Climbing Resistance/1(gradient)
  Climbing Resistance/1(F_climb [N]) -> F_climb/1, Sum1/3  "F_climb"
  Aerodynamic Resistance/1(F_aero [N]) -> F_aero/1, Sum1/1  "F_aero"
  Sum1/1 -> Sum2/1  "F_res"
  v_actual(m/s)/1 -> Rolling Resistance/1(v_actual(m/s)), Aerodynamic Resistance/1(v_desired [m/s])
  Sum2/1 -> F_drive(N)/1
  Rolling Resistance/1(F_roll [N]) -> Sum1/2, F_roll/1

== system HVModAL_Fahrzeugmodell/Vehicle_Chassis (Veh)/Interruption of Traction // Clutch ==
  F_acc[N] : Inport
  Gearchange : Inport  Port=2
  Constant1 : Constant  Value=0
  Delay3 : Delay  DelayLength=1  InitialCondition=0
  Multiport Switch : MultiPortSwitch  DataPortOrder=Zero-based contiguous  Inputs=2
  Switch : Switch  Criteria=u2 > Threshold
  veh.topology.interrupt : Constant  Value=veh.topology.interrupt
  F_acc_actual[N] : Outport
  wires:
  veh.topology.interrupt/1 -> Multiport Switch/1
  Multiport Switch/1 -> F_acc_actual[N]/1
  Constant1/1 -> Switch/3
  Gearchange/1 -> Delay3/1
  Switch/1 -> Multiport Switch/3  "Veh_v_actual"
  Delay3/1 -> Switch/2
  F_acc[N]/1 -> Multiport Switch/2, Switch/1

== system HVModAL_Fahrzeugmodell/Vehicle_Chassis (Veh)/Max Driving Force ==
  front_load [N] : Inport
  back_load [N] : Inport  Port=2
  Friction coefficient : Constant  Value=veh.wheel.coefficient_of_friction
  Gain6 : Gain  Gain=veh.wheel.radius
  Mux : Mux  Inputs=2
      settings: DisplayOption=signals
  Product : Product
  Product1 : Product
  T_wheels_max : Outport
  wires:
  Gain6/1 -> T_wheels_max/1
  Mux/1 -> Gain6/1
  front_load [N]/1 -> Product/1
  back_load [N]/1 -> Product1/1
  Friction coefficient/1 -> Product/2, Product1/2
  Product/1 -> Mux/1  "Front"
  Product1/1 -> Mux/2  "Back"

== system HVModAL_Fahrzeugmodell/Vehicle_Chassis (Veh)/Wheel Model ==
  note: Nur solange Rad haftet
  a_actual [m/s^2] : Inport
  v_wheel[m/s] : Inport  Port=2
  F_wheel [N] : Inport  Port=3
  WheelLoad [N] : Inport  Port=4
  " " : Subsystem
  F_x_wheelspin[N] : Subsystem
  Subsystem : Subsystem
  wheelspin : Subsystem
  v_actual[m/s] : Outport
  wires:
  Subsystem/1(angularVelocity[rad/s]) -> wheelspin/1(angularVelocity[rad/s]), F_x_wheelspin[N]/2(angularVelocity [rad/s])
  F_wheel [N]/1 -> F_x_wheelspin[N]/1(F_wheel [N])
  F_x_wheelspin[N]/1(F_x [N/m]) -> " "/1("F_x[N] ")
  a_actual [m/s^2]/1 -> wheelspin/3(a_actual [m/s^2])
  " "/1(wheelspin) -> wheelspin/2("wheelspin ")
  wheelspin/1(v_actual [m/s]) -> v_actual[m/s]/1
  v_wheel[m/s]/1 -> wheelspin/5(v_wheel), Subsystem/1(v_wheel [m/s])
  WheelLoad [N]/1 -> F_x_wheelspin[N]/3(wheelload), " "/2(wheelLoad[N])
  " "/2(Slip?) -> wheelspin/4(Slip?)

== system HVModAL_Fahrzeugmodell/Vehicle_Chassis (Veh)/Wheelload ==
  note: -1: front wheel drive
      | 0 : 4 wheel drive
      | 1 : back wheel drive
  Front_load [N] : Inport
  Back_load [N] : Inport  Port=2
  Drivetrain : Constant  Value=veh.wheel.drivetrain
  Multiport Switch : MultiPortSwitch  DataPortOrder=Specify indices  DataPortIndices={-1,0,1}  DiagnosticForDefault=Warning
  Wheelload [N] : Outport
  wires:
  Drivetrain/1 -> Multiport Switch/1
  Back_load [N]/1 -> Multiport Switch/4
  Front_load [N]/1 -> Multiport Switch/3, Multiport Switch/2
  Multiport Switch/1 -> Wheelload [N]/1

== system HVModAL_Fahrzeugmodell/Visualization (Vis)/Speed ==
  Bus Selector1 : BusSelector  OutputSignals=Drp_v_vehDesired
  Bus Selector2 : BusSelector  OutputSignals=Veh_v_actual
  Gain : Gain  Gain=3.6
  Gain1 : Gain  Gain=3.6
  Sum : Sum  Inputs=+-
  v_cycle(km/h) : Outport
  v_actual(km/h) : Outport  Port=2
  v_deviation(km/h) : Outport  Port=3
  wires:
  Gain1/1 -> Sum/1, v_cycle(km/h)/1  "v_cycle(km/h)"
  Gain/1 -> Sum/2, v_actual(km/h)/1  "v_actual(km/h)"
  Sum/1 -> v_deviation(km/h)/1  "v_deviation(km/h)"
  [Veh_SWBus_toworkspace] -> Bus Selector2/1
  [Drp_SWBus_toworkspace] -> Bus Selector1/1
  Bus Selector1/1 -> Gain1/1  "<Drp_v_vehDesired>"
  Bus Selector2/1 -> Gain/1  "<Veh_v_actual>"
